simulink model "scaling_signal"  (R2016b)
settings: Solver=VariableStepAuto  StartTime=0.0  StopTime=10.0  RelTol=1e-3
settings Model: Creator=momen  LastModifiedBy=momen

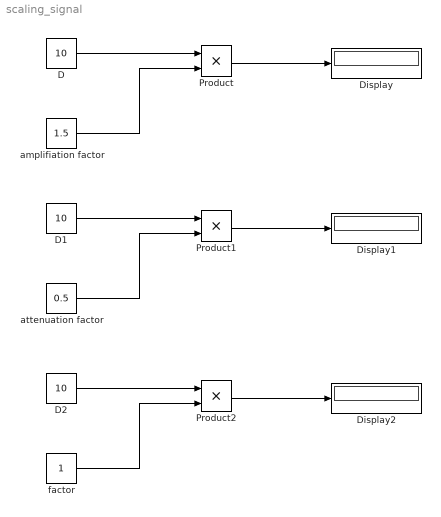
== system scaling_signal ==
  D : Constant  Value=10
  D1 : Constant  Value=10
  D2 : Constant  Value=10
  Display : Display
  Display1 : Display
  Display2 : Display
  Product : Product
  Product1 : Product
  Product2 : Product
  "amplifiation factor " : Constant  Value=1.5
  attenuation factor : Constant  Value=0.5
  factor : Constant
  wires:
  D/1 -> Product/1
  "amplifiation factor "/1 -> Product/2
  Product/1 -> Display/1
  D1/1 -> Product1/1
  attenuation factor/1 -> Product1/2
  Product1/1 -> Display1/1
  D2/1 -> Product2/1
  factor/1 -> Product2/2
  Product2/1 -> Display2/1
